simulink model "ccp_master_demo"  (Simulink 7.3)
settings: Solver=ode3  SolverMode=SingleTasking  StartTime=0.0  StopTime=10.0  RelTol=1e-3
PreLoadFcn:
  | waijung.modelPreload; % Required for working with Waijung Blockset. Do not remove.
undefined symbols (not defined in the file): LQFP48, STM32F072CB
libraries: stm32f0_can_lib x3, simulink x3, stm32f0_device_config_lib x1
(part 2 of 2)

== matlab function Embedded MATLAB Function ==
  data: rx_ready input double; Out_Tx_Enable output double; Out_Id output double; Out_Data_8 output double; Data_Update output double; rx_data8 input double; Devices_Connect output double; Temp_C output double; Humid_RH output double; Pressure_Pa output double; Light_Lux output double
function [Out_Tx_Enable, Out_Id, Out_Data_8, Data_Update,Devices_Connect, Temp_C, Humid_RH, Pressure_Pa, Light_Lux] = fcn(rx_ready, rx_data8)
%#eml


% ========================================================================
% CCP command definition
% ========================================================================
CCP_CONNECT                        = uint8(hex2dec('01'));
% CCP_GET_CCP_VERSION                = uint8(hex2dec('1B'));
% CCP_EXCHANGE_ID                    = uint8(hex2dec('17'));
% CCP_GET_SEED                       = uint8(hex2dec('12'));
% CCP_UNLOCK                         = uint8(hex2dec('13'));
% CCP_SET_MTA                        = uint8(hex2dec('02'));
% CCP_DNLOAD                         = uint8(hex2dec('03'));
% CCP_DNLOAD_6                       = uint8(hex2dec('23'));
% CCP_UPLOAD                         = uint8(hex2dec('04'));
CCP_SHORT_UP                       = uint8(hex2dec('0F'));
% CCP_SELECT_CAL_PAGE                = uint8(hex2dec('11'));
% CCP_GET_DAQ_SIZE                   = uint8(hex2dec('14'));
% CCP_SET_DAQ_PTR                    = uint8(hex2dec('15'));
% CCP_WRITE_DAQ                      = uint8(hex2dec('16'));
% CCP_START_STOP                     = uint8(hex2dec('06'));
% CCP_DISCONNECT                     = uint8(hex2dec('07'));
% CCP_SET_S_STATUS                   = uint8(hex2dec('0C'));
% CCP_GET_S_STATUS                   = uint8(hex2dec('0D'));
% CCP_BUILD_CHKSUM                   = uint8(hex2dec('0E'));
% CCP_CLEAR_MEMORY                   = uint8(hex2dec('10'));
% CCP_PROGRAM                        = uint8(hex2dec('18'));
% CCP_PROGRAM_6                      = uint8(hex2dec('22'));
% CCP_MOVE                           = uint8(hex2dec('19'));
% CCP_TEST                           = uint8(hex2dec('05'));
% CCP_GET_ACTIVE_CAL_PAGE            = uint8(hex2dec('09'));
% CCP_START_STOP_ALL                 = uint8(hex2dec('08'));
% CCP_DIAG_SERVICE                   = uint8(hex2dec('20'));
% CCP_ACTION_SERVICE                 = uint8(hex2dec('21'));

% ========================================================================
% Initial output port
% ========================================================================
MAX_SENSOR_DEVICES                 = uint8(32);
Out_Tx_Enable                      = uint8(0);
Out_Id                             = uint32(0);
Out_Data_8                         = uint8(zeros([1 8]));
Data_Update                        = uint8(0);

%persistent tmp_Devices_Connect;
persistent tmp_Temp_C; % index 0
persistent tmp_Humid_RH; % index 1
persistent tmp_Pressure_Pa; % index 2
persistent tmp_Light_Lux; % index 3

%if isempty(tmp_Devices_Connect)
%	tmp_Devices_Connect            = uint8(zeros([1 MAX_SENSOR_DEVICES]));
%end
if isempty(tmp_Temp_C)
	tmp_Temp_C                     = single(zeros([1 MAX_SENSOR_DEVICES]));
end
if isempty(tmp_Humid_RH)
	tmp_Humid_RH                   = single(zeros([1 MAX_SENSOR_DEVICES]));
end
if isempty(tmp_Pressure_Pa)
	tmp_Pressure_Pa                = single(zeros([1 MAX_SENSOR_DEVICES]));
end
if isempty(tmp_Light_Lux)
	tmp_Light_Lux                  = single(zeros([1 MAX_SENSOR_DEVICES]));
end

% ========================================================================
% Operation state/ var
% ========================================================================
RX_TIMEOUT_COUNT = uint8(5);

OP_STATE_CONNECTION = uint8(0);
OP_STATE_READ_VALUES= uint8(1);

% Sensors reading state
persistent sensors_reading_index;
persistent sensors_reading_state;
if isempty(sensors_reading_index)
	sensors_reading_index = uint8(0);
end
if isempty(sensors_reading_state)
	sensors_reading_state = uint8(0);
end

% Device connection list
persistent Connection_Status_List;
if isempty(Connection_Status_List)
	Connection_Status_List         = uint8(zeros([1 MAX_SENSOR_DEVICES]));
end

% State index
persistent psOperation_State_Index;
if isempty(psOperation_State_Index)
	psOperation_State_Index = uint8(0);
end
% On Enter state event
persistent psOperation_State_OnEnter;
if isempty(psOperation_State_OnEnter)
	psOperation_State_OnEnter = uint8(1);
end
% Device index
persistent psOperation_Device_Index;
if isempty(psOperation_Device_Index)
	psOperation_Device_Index = uint8(0);
end
% Timeout status
persistent psOperation_Timeout_Status;
if isempty(psOperation_Timeout_Status);
	psOperation_Timeout_Status = uint8(0);
end
% Timeout counter
persistent psOperation_Timeout_Counter;
if isempty(psOperation_Timeout_Counter)
	psOperation_Timeout_Counter = uint8(0);
end

% Connection state
persistent psConnection_State;
if isempty(psConnection_State)
	psConnection_State = uint8(0);
end

% Determine OnEnter Status flag
tmp_state_index = psOperation_State_Index;

% Operation state
switch tmp_state_index
	% --- CONNECT ---
	case OP_STATE_CONNECTION
		if (psOperation_State_OnEnter ~= uint8(0))
			% Reset device ID
			psOperation_Device_Index = uint8(0);
			% Clear timeout
			psOperation_Timeout_Counter = uint8(0);
			psOperation_Timeout_Status = uint8(0);	
			
			psConnection_State = uint8(0);
		end
		
		% Transmit
		if psConnection_State == uint8(0)
			% Transmit connection command every Ts sec (10ms).
			if (psOperation_Device_Index < MAX_SENSOR_DEVICES)
				Out_Data_8(1) = CCP_CONNECT; % Command
				Out_Data_8(2) = psOperation_Device_Index; % CTR
				Out_Id = uint32(psOperation_Device_Index); % CAN ID
				Out_Tx_Enable = uint8(1); % Enable Tx
				
				% Goto wait for response
				psConnection_State = uint8(1);
				% Clear timeout
				psOperation_Timeout_Counter = uint8(0);
				psOperation_Timeout_Status = uint8(0);
			else
				% Change state
				tmp_state_index = tmp_state_index + uint8(1);
			end
		% Receive
		else
			next_id = false;
			% Check received CAN packet
			if rx_ready ~= uint8(0)
				if (rx_data8(1) == uint8(255)) && (rx_data8(2) == uint8(0)) && (rx_data8(3) <MAX_SENSOR_DEVICES)
					idx = rx_data8(3) + uint8(1); % 1 Base indexnig
					Connection_Status_List(idx) = uint8(1);
					
					next_id = true;
				end
			end
			% Timeout check
			if psOperation_Timeout_Counter < RX_TIMEOUT_COUNT
				psOperation_Timeout_Counter = psOperation_Timeout_Counter + uint8(1);
			else
				Connection_Status_List(psOperation_Device_Index+1) = uint8(0);
				next_id = true;
			end
			% Data receive or timeout 
			if next_id
				psOperation_Device_Index = psOperation_Device_Index + uint8(1);
				psConnection_State = uint8(0);
			end
		end

	% --- READING ---
	case OP_STATE_READ_VALUES
		if (psOperation_State_OnEnter ~= uint8(0)) % OnEnter
			% Reset device ID
			psOperation_Device_Index = uint8(0);
			% Clear timeout
			psOperation_Timeout_Counter = uint8(0);
			psOperation_Timeout_Status = uint8(0);
			% Reading state
			sensors_reading_index = uint8(0);
			sensors_reading_state = uint8(0);
		end
		% Command
		if sensors_reading_state == uint8(0) % Initiate
			if psOperation_Device_Index >= MAX_SENSOR_DEVICES
				psOperation_Device_Index = uint8(0); % Reset device index
				sensors_reading_index = sensors_reading_index + uint8(1);
				if sensors_reading_index >= 4 % Number of meas values
					tmp_state_index = uint8(0); % Re-connect
					sensors_reading_index = uint8(0); % Reset reading index
					Data_Update = uint8(1); % Indicate the data is ready for use
				end
			end
			% Transmit command
			idx = psOperation_Device_Index + uint8(1);
			if Connection_Status_List(idx) ~= uint8(0)
				Out_Data_8(1) = CCP_SHORT_UP; % Command
				Out_Data_8(2) = psOperation_Device_Index; % CTR
				Out_Data_8(3) = uint8(4); % Size
				Out_Data_8(4) = uint8(1); % Ext, RO memory
				Out_Data_8(5) = uint8(0); % Addr A3
				Out_Data_8(6) = uint8(0); % Addr A2
				Out_Data_8(7) = uint8(0); % Addr A1
				Out_Data_8(8) = uint8(sensors_reading_index*4); % Addr A0
				
				Out_Id = uint32(psOperation_Device_Index); % CAN ID
				Out_Tx_Enable = uint8(1); % Enable Tx
				
				% Clear timeout
				psOperation_Timeout_Counter = uint8(0);
				psOperation_Timeout_Status = uint8(0);
			
				% Go to wait for response
				sensors_reading_state = sensors_reading_state + uint8(1);
			else
				% Current index is not connected
				psOperation_Device_Index = psOperation_Device_Index + uint8(1);
			end
		% Response
		else
			intiate = false;
			% Data Ready ?
			if (rx_ready ~= uint8(0)) && (rx_data8(1) == uint8(255)) && (rx_data8(2) == uint8(0)) && (rx_data8(3) == psOperation_Device_Index)
				tmp = uint32(rx_data8(4)) ...
					+ uint32(uint32(rx_data8(5))*uint32(hex2dec('100'))) ...
					+ uint32(uint32(rx_data8(6))*uint32(hex2dec('10000'))) ...
					+ uint32(uint32(rx_data8(7))*uint32(hex2dec('1000000')));
				
				switch sensors_reading_index
					case 0
						tmp_Temp_C (psOperation_Device_Index + 1) = single(tmp)/single(256);
					case 1
						tmp_Humid_RH (psOperation_Device_Index + 1) = single(tmp)/single(256);						
					case 2
						tmp_Pressure_Pa (psOperation_Device_Index + 1) = single(tmp)/single(4);
					case 3
						tmp_Light_Lux (psOperation_Device_Index + 1) = single(tmp)/single(4);
				end
				intiate = true;
				
				% Clear timeout
				psOperation_Timeout_Counter = uint8(0);
				psOperation_Timeout_Status = uint8(0);				
			else
				% Timeout check
				if psOperation_Timeout_Counter > 20 % 200ms
					Connection_Status_List(psOperation_Device_Index) = uint8(0); % Deactivate connection for active index
					intiate = true;
				else
					psOperation_Timeout_Counter = psOperation_Timeout_Counter + uint8(1);
				end
			end
			
			% Back to initiate state
			if intiate
				sensors_reading_state = uint8(0); % Initiate
				psOperation_Device_Index = psOperation_Device_Index + uint8(1);
			end
		end
	otherwise
end

% ========================================================================
if tmp_state_index ~= psOperation_State_Index
	% Set OnEnter
	psOperation_State_OnEnter = uint8(1);
	% Update operation state
	psOperation_State_Index = tmp_state_index;
else
	% Clear OnEnter
	psOperation_State_OnEnter = uint8(0);
end

% ========================================================================
% Update output port
% ========================================================================
Devices_Connect = Connection_Status_List;%tmp_Devices_Connect;
Temp_C = tmp_Temp_C;
Humid_RH = tmp_Humid_RH;
Pressure_Pa = tmp_Pressure_Pa;
Light_Lux = tmp_Light_Lux;
